simulink model "classmodel1"  (R2023a)
settings: Solver=VariableStepAuto  StartTime=0.0  StopTime=50  RelTol=1e-3
libraries: Solver_SF x2, simulink_extras x2, simulink x1
settings Model: Creator=Jessie  LastModifiedBy=Jessie

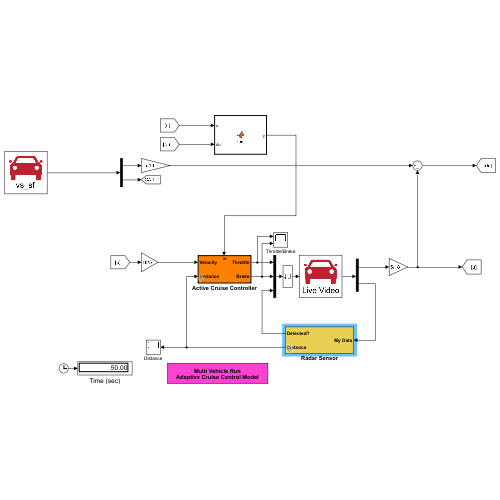
[thumbnail: Simulink's stored preview of the top-level diagram]
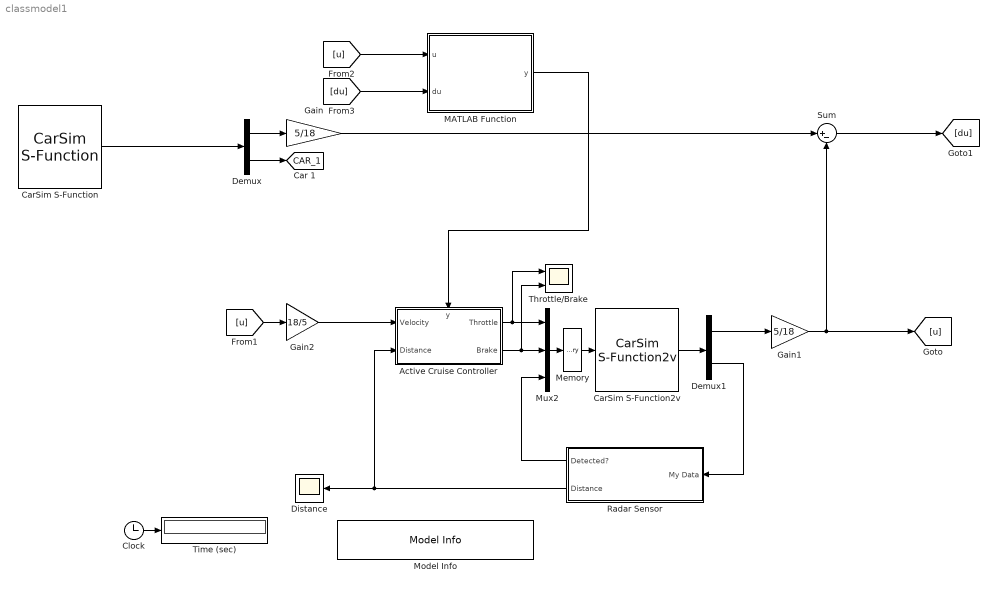
== system classmodel1 ==
  Active Cruise Controller : Subsystem  TreatAsAtomicUnit=on  mask{VX=95, DISTANCE=50}
      mask prompts: VX "Setup Velocity (km/h)"; DISTANCE "Setup Distance (m)"
      settings: PortSchema="{\"entries\":[{\"content\":{\"sides\":[{\"content\":{\"connectorIds\":[\"In1\",\"In2\"]},\"type\":\"ConnectorPlacement.EquallySpacedRectSide\",\"uuid\":\"a707c70e-71f4-4fb5-a959-dbfc8f6ff7b8\"},{\"content\":{\"connectorIds\":[\"Out1\",\"Out2\"],\"side\":\"RIGHT\"},\"type\":\"ConnectorPlacement.EquallySpacedRectSide\",\"uuid\":\"2085ab1f-b221-4f19-b8db-30e0e9abc42f\"},{\"content\":{\"connectorIds\":[\"In3\"],\"side\":\"TOP\"},\"type\":\"ConnectorPlacement.EquallySpacedRectSide\",\"uuid\":\"5e354b9b-478a-4a26-a8ee-0ced1ca5ae7f\"}]},\"type\":\"ConnectorPlacement.EquallySpacedConnector\",\"uuid\":\"3215cfc1-7083-47aa-be94-4e92c175cccd\"}],\"packageUris\":[\"http://schema.mathworks.com/mf0/Connector/R2020b\"],\"version\":\"1.0\"}"
      mask DialogControl ParameterGroupVar Prompt: 参数
  CarSim S-Function : Solver_SF/CarSim S-Function  Priority=1  SIMFILE=Radar_Acc_ExtSen_Car_1.sim
  CarSim S-Function2v : Solver_SF/CarSim S-Function2v  Priority=1  SIMFILE=Radar_Acc_ExtSen_Car_2.sim
      settings: SourceProductName=CarSim S-Function
  Clock : Clock
  Demux : Demux  Outputs=[1 3]
      settings: DisplayOption=none
  Demux1 : Demux  Outputs=[1 3]
      settings: DisplayOption=none
  Distance : Scope
  Gain : Gain  Gain=5/18
  Gain1 : Gain  Gain=5/18
  Gain2 : Gain  Gain=18/5
  MATLAB Function : MATLAB Function  TreatAsAtomicUnit=on
  Memory : Memory  InheritSampleTime=on
  Model Info : simulink/Model-Wide Utilities/Model Info  Frame=on  DisplayStringWithTags=Multi Vehicle Run Adaptive Cruise Control Model  HorizontalTextAlignment=Center  LeftAlignmentValue=0.5
  Mux2 : Mux  Inputs=3
  Radar Sensor : Subsystem  mask{S_ANGLE=10, S_DISTANCE=70}
      mask prompts: S_ANGLE "View Angle (deg)"; S_DISTANCE "Distance Range (m)"
      mask help:
      | An example of a radar sensor. It can detect the distance between the sensor and another object according its position (Xo, Yo).
      |
      | Input parameters are View Angle(deg) and radar detectable distance(m).
      mask init:
      | d_ang= str2double(S_ANGLE)/2;
      | set_param([gcb '/View Angle'], 'Threshold', sprintf('%0.2f', d_ang));
      | set_param([gcb '/L-Radar'], 'Value', S_DISTANCE);
  Sum : Sum  Inputs=|+-
  Throttle/Brake : Scope  NumInputPorts=2
  Time (sec) : Display
      settings: Format=bank  Decimation=100
  tag scope: CAR_1=global
  wires:
  CarSim S-Function2v/1 -> Demux1/1
  Radar Sensor/1(Detected?) -> Mux2/3
  Mux2/1 -> Memory/1
  Demux1/1 -> Gain1/1
  CarSim S-Function/1 -> Demux/1
  Demux/1 -> Gain/1
  Radar Sensor/2(Distance) -> Distance/1, Active Cruise Controller/2(Distance)
  Clock/1 -> Time (sec)/1
  Active Cruise Controller/1(Throttle) -> Mux2/1, Throttle/Brake/1
  Demux/2 -> [CAR_1]
  Demux1/2 -> Radar Sensor/1(My Data)
  Active Cruise Controller/2(Brake) -> Mux2/2, Throttle/Brake/2
  Gain/1 -> Sum/1
  Gain1/1 -> Sum/2, [u]
  Sum/1 -> [du]
  Memory/1 -> CarSim S-Function2v/1
  Gain2/1 -> Active Cruise Controller/1(Velocity)
  [u] -> Gain2/1
  [du] -> MATLAB Function/2(du)
  [u] -> MATLAB Function/1(u)
  MATLAB Function/1(y) -> Active Cruise Controller/3(y)

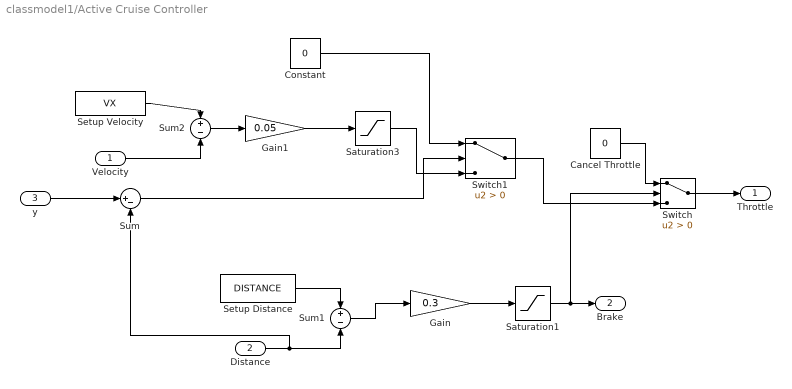
== system classmodel1/Active Cruise Controller ==
  Velocity : Inport
  Distance : Inport  Port=2
  y : Inport  Port=3
  Cancel Throttle : Constant  Value=0
  Constant : Constant  Value=0
  Gain : Gain  Gain=0.3  SaturateOnIntegerOverflow=on  OutDataTypeStr=Inherit: Same as input  ParamDataTypeStr=Inherit: Same as input
  Gain1 : Gain  Gain=0.05  SaturateOnIntegerOverflow=on  OutDataTypeStr=Inherit: Same as input  ParamDataTypeStr=Inherit: Same as input
  Saturation1 : Saturate  UpperLimit=15  LowerLimit=0
  Saturation3 : Saturate  UpperLimit=1  LowerLimit=0
  Setup Distance : Constant  Value=DISTANCE
  Setup Velocity : Constant  Value=VX
  Sum : Sum  Inputs=|+-
  Sum1 : Sum  Inputs=+-  InputSameDT=on  SaturateOnIntegerOverflow=on  OutDataTypeStr=Inherit: Same as first input
  Sum2 : Sum  Inputs=+-  InputSameDT=on  SaturateOnIntegerOverflow=on  OutDataTypeStr=Inherit: Same as first input
  Switch : Switch  Criteria=u2 > Threshold  InputSameDT=off
  Switch1 : Switch  Criteria=u2 > Threshold  SaturateOnIntegerOverflow=off  InputSameDT=off
  Throttle : Outport
  Brake : Outport  Port=2
  wires:
  Gain/1 -> Saturation1/1
  Saturation1/1 -> Brake/1, Switch/2
  Setup Velocity/1 -> Sum2/1
  Sum2/1 -> Gain1/1
  Gain1/1 -> Saturation3/1
  Velocity/1 -> Sum2/2
  Switch/1 -> Throttle/1
  Setup Distance/1 -> Sum1/1
  Distance/1 -> Sum1/2, Sum/2
  Sum1/1 -> Gain/1
  Cancel Throttle/1 -> Switch/1
  Saturation3/1 -> Switch1/3
  Constant/1 -> Switch1/1
  y/1 -> Sum/1
  Sum/1 -> Switch1/2
  Switch1/1 -> Switch/3

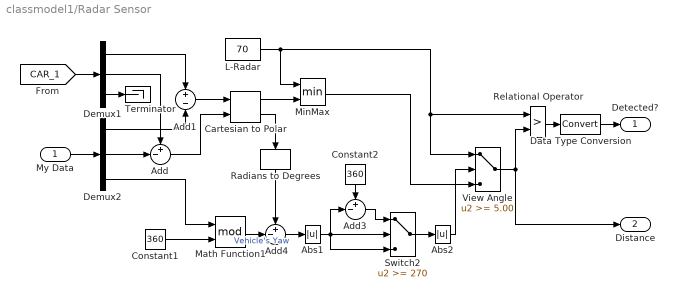
== system classmodel1/Radar Sensor ==
  My Data : Inport
  Abs1 : Abs  SaturateOnIntegerOverflow=off
  Abs2 : Abs  SaturateOnIntegerOverflow=off
  Add : Sum  Inputs=+-|
  Add1 : Sum  Inputs=+-
  Add3 : Sum  Inputs=+-|
  Add4 : Sum  Inputs=+-|
  Cartesian to Polar : simulink_extras/Transformations/Cartesian to Polar
  Constant1 : Constant  Value=360
  Constant2 : Constant  Value=360
  Data Type Conversion : DataTypeConversion  SaturateOnIntegerOverflow=off
  Demux1 : Demux  Outputs=3
      settings: DisplayOption=none
  Demux2 : Demux  Outputs=3
      settings: DisplayOption=none
  L-Radar : Constant  Value=70
  Math Function1 : Math  Operator=mod  SignedPower=on
  MinMax : MinMax  Inputs=2  InputSameDT=on  SaturateOnIntegerOverflow=on
  Radians to Degrees : simulink_extras/Transformations/Radians to Degrees
  Relational Operator : RelationalOperator  Operator=>  OutDataTypeStr=boolean  InputSameDT=off
  Switch2 : Switch  Threshold=270  SaturateOnIntegerOverflow=off  InputSameDT=off
  Terminator : Terminator
  View Angle : Switch  Threshold=5.00  SaturateOnIntegerOverflow=off  InputSameDT=off
  Detected? : Outport
  Distance : Outport  Port=2
  wires:
  Demux2/3 -> Math Function1/1
  Constant1/1 -> Math Function1/2
  Add/1 -> Cartesian to Polar/2
  Add1/1 -> Cartesian to Polar/1
  Demux2/1 -> Add1/2
  Demux1/1 -> Add1/1
  Demux2/2 -> Add/2
  Demux1/2 -> Add/1
  Demux1/3 -> Terminator/1
  My Data/1 -> Demux2/1
  [CAR_1] -> Demux1/1
  Math Function1/1 -> Add4/2  "Vehicle's Yaw"
  Add4/1 -> Abs1/1
  Abs1/1 -> Switch2/2, Add3/2, Switch2/3
  Add3/1 -> Switch2/1
  Constant2/1 -> Add3/1
  L-Radar/1 -> MinMax/1, View Angle/1, Relational Operator/1
  MinMax/1 -> View Angle/3
  Switch2/1 -> Abs2/1
  Abs2/1 -> View Angle/2
  View Angle/1 -> Distance/1, Relational Operator/2
  Relational Operator/1 -> Data Type Conversion/1
  Data Type Conversion/1 -> Detected?/1
  Radians to Degrees/1 -> Add4/1
  Cartesian to Polar/1 -> MinMax/2
  Cartesian to Polar/2 -> Radians to Degrees/1

== matlab function classmodel1/MATLAB Function ==
  data: u input; y output; du input
function y = fcn(u,du)
Th=1.5;
K1=0.425;
d0=3;
y = Th*u-K1*du+d0;
